simulink model "baitap"  (R2015b)
settings: Solver=VariableStepAuto  StartTime=0.0  StopTime=10.0  RelTol=1e-3
settings Model: Creator=Chinh  LastModifiedBy=Chinh

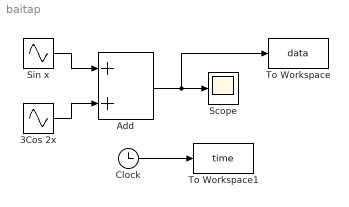
== system baitap ==
  3Cos 2x : Sin  Amplitude=3  Frequency=2  Phase=pi/2  SampleTime=0
  Add : Sum
  Clock : Clock
      settings: Decimation=100
  Scope : Scope
  Sin x : Sin  SampleTime=0
  To Workspace : ToWorkspace  VariableName=data  SampleTime=-1
  To Workspace1 : ToWorkspace  VariableName=time  SampleTime=-1
  wires:
  Sin x/1 -> Add/1
  3Cos 2x/1 -> Add/2
  Add/1 -> To Workspace/1, Scope/1
  Clock/1 -> To Workspace1/1
